simulink model "adcs_model"  (R2024b)
settings: Solver=ode4  StartTime=0.0  StopTime=p.t_final  FixedStep=p.dt  RelTol=1e-3
values from neighbouring files (symbols this model uses):
  p = adcs_params()    [run_simulink.m]
settings Model: Creator=ricca  LastModifiedBy=ricca

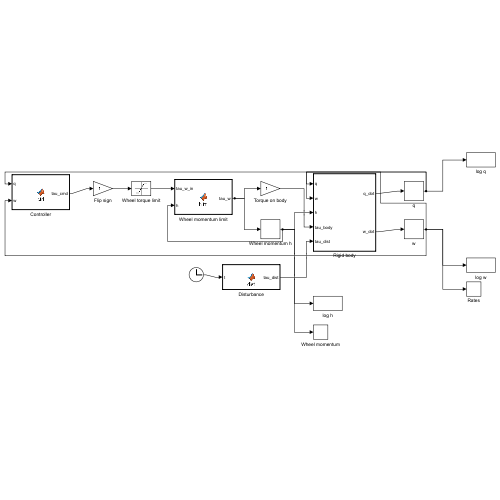
[thumbnail: Simulink's stored preview of the top-level diagram]
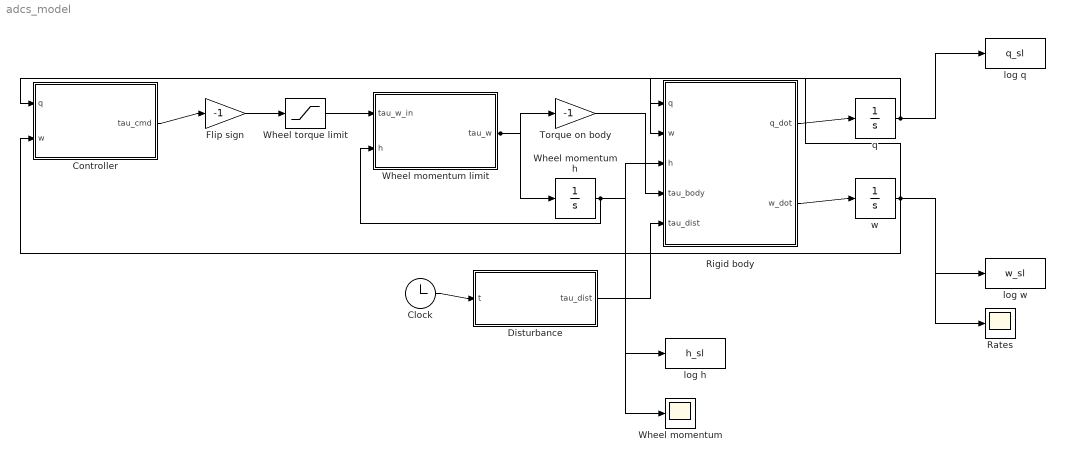
== system adcs_model ==
  Clock : Clock
  Controller : MATLAB Function  TreatAsAtomicUnit=on
  Disturbance : MATLAB Function  TreatAsAtomicUnit=on
  Flip sign : Gain  Gain=-1
  Rates : Scope
  Rigid body : MATLAB Function  TreatAsAtomicUnit=on
  Torque on body : Gain  Gain=-1
  Wheel momentum : Scope
  Wheel momentum h : Integrator  InitialCondition=zeros(3,1)
  Wheel momentum limit : MATLAB Function  TreatAsAtomicUnit=on
  Wheel torque limit : Saturate  UpperLimit=p.tau_max  LowerLimit=-p.tau_max
  log h : ToWorkspace  VariableName=h_sl  SampleTime=-1
  log q : ToWorkspace  VariableName=q_sl  SampleTime=-1
  log w : ToWorkspace  VariableName=w_sl  SampleTime=-1
  q : Integrator  InitialCondition=p.q0
  w : Integrator  InitialCondition=p.w0
  wires:
  Controller/1(tau_cmd) -> Flip sign/1
  Flip sign/1 -> Wheel torque limit/1
  Wheel torque limit/1 -> Wheel momentum limit/1(tau_w_in)
  Wheel momentum limit/1(tau_w) -> Wheel momentum h/1, Torque on body/1
  Wheel momentum h/1 -> Wheel momentum limit/2(h), Rigid body/3(h), log h/1, Wheel momentum/1
  Torque on body/1 -> Rigid body/4(tau_body)
  Clock/1 -> Disturbance/1(t)
  Disturbance/1(tau_dist) -> Rigid body/5(tau_dist)
  Rigid body/1(q_dot) -> q/1
  Rigid body/2(w_dot) -> w/1
  q/1 -> log q/1, Controller/1(q), Rigid body/1(q)
  w/1 -> log w/1, Rates/1, Controller/2(w), Rigid body/2(w)

== matlab function adcs_model/Wheel momentum limit ==
  data: tau_w_in input; tau_w output; h input; p parameter
function tau_w = hlim(tau_w_in, h, p)
% if a wheel is full it cannot be pushed further the same way
% (same rule as reaction_wheels.m)
tau_w = tau_w_in;
for i = 1:3
    if abs(h(i)) >= p.h_max && sign(tau_w(i)) == sign(h(i))
        tau_w(i) = 0;
    end
end

== matlab function adcs_model/Controller ==
  data: q input; tau_cmd output; w input; p parameter
function tau_cmd = ctrl(q, w, p)
% same PD with capped slew rate as simulate_adcs.m, but with the TRUE q and w
qe = quat_error(p.q_ref, q / norm(q));
w_cmd = -(p.Kp / p.Kd) * qe(2:4);
if norm(w_cmd) > p.w_max
    w_cmd = w_cmd / norm(w_cmd) * p.w_max;
end
tau_cmd = -p.Kd * (w - w_cmd);

== matlab function adcs_model/Disturbance ==
  data: t input; tau_dist output; p parameter
function tau_dist = dist(t, p)
tau_dist = disturbance_torque(t, p);

== matlab function adcs_model/Rigid body ==
  data: q input; q_dot output; w input; h input; tau_body input; tau_dist input; w_dot output; p parameter
function [q_dot, w_dot] = body(q, w, h, tau_body, tau_dist, p)
% Euler equation with the wheel momentum, and quaternion kinematics
q = q / norm(q);
w_dot = p.I \ (-cross(w, p.I*w + h) + tau_body + tau_dist);
q_dot = 0.5 * quat_mult(q, [0; w]);
